simulink model "coolcats"  (R2019b)
settings: Solver=VariableStepAuto  StartTime=0.0  StopTime=70  MaxStep=1e-4  RelTol=1e-3
values from neighbouring files (symbols this model uses):
  Beff = bm3 + bg4    (= 4.60621556139e-05)    [controller.m]
  g = -9.8    [controller.m]
  Jb = 2/5*(Rb^2)*m    (= 1.340328e-06)    [controller.m]
  Jeff = Jm3 + Jload / (N^2)    (= 2.25012674867e-07)    [controller.m]
  KE = KE3    (= 0.00733386)    [controller.m]
  KS = 10    [controller.m]
  KT = KT3    (= 0.00733)    [controller.m]
  L = L3    (= 3.5e-05)    [controller.m]
  m = 0.0335082    [controller.m]
  N = 200    [controller.m]
  r = 6e-3    (= 0.006)    [controller.m]
  R = R3    (= 1.3)    [controller.m]
libraries: simulink x2
settings Model: Creator=spenc  LastModifiedBy=zlink
settings DataIOCC: ReturnWorkspaceOutputs=off
settings DebuggingCC: ArithmeticOperatorsInVariantConditions=warning
settings SFSimCC: SimUseLocalCustomCode=off  CustomCodeUndefinedFunction=UseInterfaceOnly
settings RTWCC: RTWUseLocalCustomCode=off

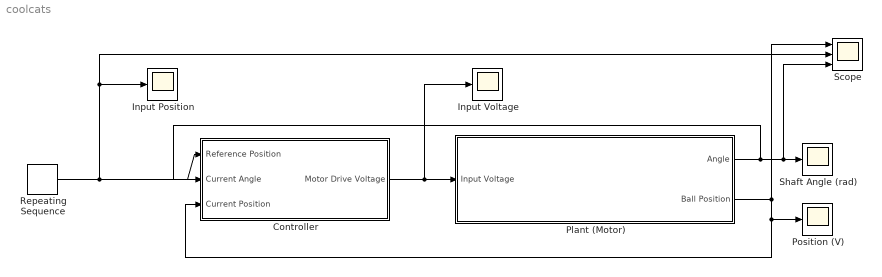
== system coolcats ==
  Controller : Subsystem
  Input Position : Scope
  Input Voltage : Scope
  Plant (Motor) : Subsystem
  Position (V) : Scope
  Repeating Sequence : simulink/Sources/Repeating Sequence  rep_seq_t=[0 1 1.01 2 2.01 3 3.01 4 4.01 5 5.01 6 6.01 7] * 10  rep_seq_y=[5 5 15 15 -20 -20 10 10 0 0 20 20 -20 -20]
  Scope : Scope  NumInputPorts=3
  Shaft Angle (rad) : Scope
  wires:
  Plant (Motor)/1(Angle) -> Controller/2(Current Angle), Scope/3, Shaft Angle (rad)/1
  Repeating Sequence/1 -> Controller/1(Reference Position), Scope/2, Input Position/1
  Plant (Motor)/2(Ball Position) -> Scope/1, Position (V)/1, Controller/3(Current Position)
  Controller/1(Motor Drive Voltage) -> Plant (Motor)/1(Input Voltage), Input Voltage/1

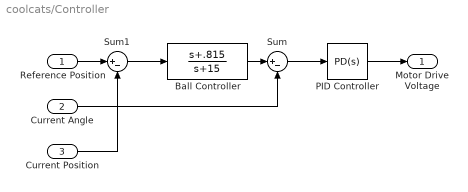
== system coolcats/Controller ==
  Reference Position : Inport
  Current Angle : Inport  Port=2
  Current Position : Inport  Port=3
  Ball Controller : TransferFcn  Numerator=[1 .815]  Denominator=[1 15]
  PID Controller : simulink/Continuous/PID Controller  Controller=PD  Form=Parallel  TimeDomain=Continuous-time  SampleTime=-1  IntegratorMethod=Forward Euler  FilterMethod=Forward Euler  ControllerParametersSource=internal  P=2000  I=1  D=10  UseFilter=on  N=100000  TunerSelectOption=Transfer Function Based (PID Tuner App)  InitialConditionSource=internal  InitialConditionForIntegrator=0  InitialConditionForFilter=0  DifferentiatorICPrevScaledInput=0  ExternalReset=none  TrackingMode=off  Kt=1  LimitOutput=on  UpperSaturationLimit=6  LowerSaturationLimit=-6  LinearizeAsGain=on  AntiWindupMode=none  Kb=1  POutMin=[]  POutMax=[]  IOutMin=[]  IOutMax=[]  DOutMin=[]  DOutMax=[]  NOutMin=[]  NOutMax=[]  SumOutMin=[]  SumOutMax=[]  SaturationOutMin=[]  SaturationOutMax=[]  PParamMin=[]  PParamMax=[]  IParamMin=[]  IParamMax=[]  DParamMin=[]  DParamMax=[]  NParamMin=[]  NParamMax=[]  KbParamMin=[]  KbParamMax=[]  KtParamMin=[]  KtParamMax=[]  KbOutMin=[]  KbOutMax=[]  KtOutMin=[]  KtOutMax=[]  IntegratorOutMin=[]  IntegratorOutMax=[]  FilterOutMin=[]  FilterOutMax=[]  SumI1OutMin=[]  SumI1OutMax=[]  SumI2OutMin=[]  SumI2OutMax=[]  SumI3OutMin=[]  SumI3OutMax=[]  SumI4OutMin=[]  SumI4OutMax=[]  SumDOutMin=[]  SumDOutMax=[]  DifferentiatorOutMin=[]  DifferentiatorOutMax=[]  FilterDiffOutCoefMin=[]  FilterDiffOutCoefMax=[]  ReciprocalOutMin=[]  ReciprocalOutMax=[]  SumDenOutMin=[]  SumDenOutMax=[]  SumNumOutMin=[]  SumNumOutMax=[]  DivideOutMin=[]  DivideOutMax=[]  IntegratorContinuousStateAttributes=''  IntegratorStateMustResolveToSignalObject=off  IntegratorRTWStateStorageClass=Auto  FilterContinuousStateAttributes=''  FilterStateMustResolveToSignalObject=off  FilterRTWStateStorageClass=Auto  ParallelPVariant=InternalParameters  IdealPVariant=Disabled  IVariant=Disabled  DVariant=InternalParameters  IntegratorVariant=Disabled  SatVariant=Enabled  AWVariant=Disabled  PCopyVariant=Disabled  TRVariant=Disabled  FdbkBlocksVariant=Forward  IdealPFdbkVariant=Disabled  SatFdbkVariant=Disabled  DerivativeFilterVariant=ContFilter  NVariant=InternalParameters  NCopyVariant=Disabled  FilterICVariant=InternalICsFilter  IntegratorICVariant=Disabled  ExternalResetVariant=Disabled  TRSumVariant=Passthrough  SumFdbkVariant=Disabled  SumVariant=Sum_PD
  Sum : Sum  Inputs=|+-
  Sum1 : Sum  Inputs=|+-
  Motor Drive Voltage : Outport
  wires:
  Current Angle/1 -> Sum/2
  Current Position/1 -> Sum1/2
  Reference Position/1 -> Sum1/1
  Sum/1 -> PID Controller/1
  Sum1/1 -> Ball Controller/1
  Ball Controller/1 -> Sum/1
  PID Controller/1 -> Motor Drive Voltage/1

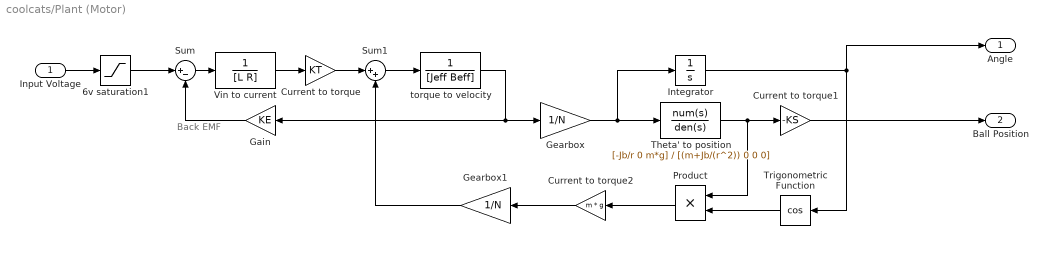
== system coolcats/Plant (Motor) ==
  note: Back EMF
  Input Voltage : Inport
  6v saturation1 : Saturate  UpperLimit=6  LowerLimit=-6
  Current to torque : Gain  Gain=KT
  Current to torque1 : Gain  Gain=-KS
  Current to torque2 : Gain  Gain=m * g
  Gain : Gain  Gain=KE
  Gearbox : Gain  Gain=1/N
  Gearbox1 : Gain  Gain=1/N
  Integrator : Integrator
  Product : Product
  Sum : Sum  Inputs=|+-
  Sum1 : Sum  Inputs=|++
  Theta' to position : TransferFcn  Numerator=[-Jb/r 0 m*g]  Denominator=[(m+Jb/(r^2)) 0 0 0]
  Trigonometric Function : Trigonometry  Operator=cos
  Vin to current : TransferFcn  Denominator=[L R]
  torque to velocity : TransferFcn  Numerator=1  Denominator=[Jeff Beff]
  Angle : Outport
  Ball Position : Outport  Port=2
  wires:
  Gain/1 -> Sum/2
  Integrator/1 -> Angle/1, Trigonometric Function/1
  torque to velocity/1 -> Gearbox/1, Gain/1
  Theta' to position/1 -> Product/1, Current to torque1/1
  Current to torque/1 -> Sum1/1
  Gearbox/1 -> Integrator/1, Theta' to position/1
  Trigonometric Function/1 -> Product/2
  Input Voltage/1 -> 6v saturation1/1
  Sum/1 -> Vin to current/1
  Vin to current/1 -> Current to torque/1
  6v saturation1/1 -> Sum/1
  Sum1/1 -> torque to velocity/1
  Product/1 -> Current to torque2/1
  Gearbox1/1 -> Sum1/2
  Current to torque2/1 -> Gearbox1/1
  Current to torque1/1 -> Ball Position/1
